simulink library "GaitGenerator"  (R2016b)
settings: Solver=VariableStepAuto  StartTime=0.0  StopTime=10.0  RelTol=1e-3
libraries: lookUpTable x7
settings Model: Creator=Nathan  LastModifiedBy=lucadelaat

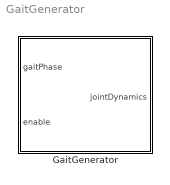
== system GaitGenerator ==
  GaitGenerator : Subsystem

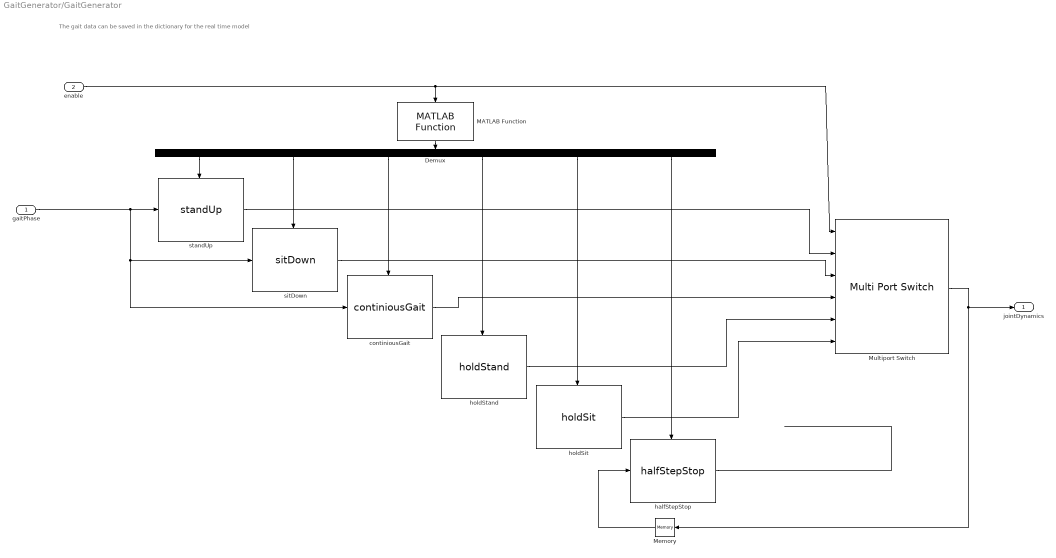
== system GaitGenerator/GaitGenerator ==
  note: The gait data can be saved in the dictionary for the real time model
  gaitPhase : Inport
  enable : Inport  Port=2
  Demux : Demux  Outputs=6
  MATLAB Function : lookUpTable/GaitGenerator/MATLAB Function
  Memory : Memory
  Multiport Switch : MultiPortSwitch  DataPortOrder=Specify indices  Inputs=4  DataPortIndices={ExoskeletonState.STANDINGUP,ExoskeletonState.SITTINGDOWN,ExoskeletonState.CONTINUOUSGAIT,ExoskeletonState.HOLDSTAND,ExoskeletonState.HOLDSIT}
  continiousGait : lookUpTable/GaitGenerator/continiousGait
  halfStepStop : lookUpTable/GaitGenerator/halfStepStop
  holdSit : lookUpTable/GaitGenerator/holdSit
  holdStand : lookUpTable/GaitGenerator/holdStand
  "sitDown " : lookUpTable/GaitGenerator/sitDown 
  standUp : lookUpTable/GaitGenerator/standUp
  jointDynamics : Outport  OutDataTypeStr=Bus: JointDynamics
  wires:
  "sitDown "/1 -> Multiport Switch/3
  Demux/4 -> holdStand/Enable
  Demux/3 -> continiousGait/Enable
  Demux/2 -> "sitDown "/Enable
  enable/1 -> Multiport Switch/1, MATLAB Function/1
  standUp/1 -> Multiport Switch/2
  holdStand/1 -> Multiport Switch/5
  Multiport Switch/1 -> Memory/1, jointDynamics/1
  continiousGait/1 -> Multiport Switch/4
  gaitPhase/1 -> standUp/1, continiousGait/1, "sitDown "/1
  Demux/1 -> standUp/Enable
  MATLAB Function/1 -> Demux/1
  Demux/5 -> holdSit/Enable
  holdSit/1 -> Multiport Switch/6
  halfStepStop/1 -> ?
  Memory/1 -> halfStepStop/1
  Demux/6 -> halfStepStop/Enable
